simulink model "flat_model"  (R2023a)
settings: Solver=ode45  StartTime=0.0  StopTime=10.0  RelTol=1e-3  EnableMultiTasking=on
undefined symbols (not defined in the file): a0x, a0y, a0z, a1x, a1y, a1z, g, m
settings Model: Creator=Cesar Mtz  LastModifiedBy=20808
settings SolverCC: AlgebraicLoopSolver=TrustRegion
settings DataIOCC: LimitDataPoints=on  SaveFormat=Array  SignalLoggingSaveFormat=ModelDataLogs  ReturnWorkspaceOutputs=off
settings OptimizationCC: ExpressionDepthLimit=2147483647  LifeSpan=inf
settings DebuggingCC: UnderspecifiedInitializationDetection=Classic  MergeDetectMultiDrivingBlocksExec=none  SolverPrmCheckMsg=warning  FcnCallInpInsideContextMsg=warning  UnconnectedInputMsg=warning  UnconnectedOutputMsg=warning  UnconnectedLineMsg=warning  StateNameClashWarn=warning  SFUnexpectedBacktrackingDiag=warning  SFNoUnconditionalDefaultTransitionDiag=warning  SFExecutionAtInitializationDiag=none  ArithmeticOperatorsInVariantConditions=warning
settings HardwareCC: ProdBitPerPointer=32  ProdBitPerSizeT=32  ProdBitPerPtrDiffT=32  ProdLargestAtomicFloat=None  ProdIntDivRoundTo=Undefined  ProdEndianess=Unspecified  ProdWordSize=32  ProdHWDeviceType=32-bit Generic
settings ModelReferenceCC: EnableRefExpFcnMdlSchedulingChecks=on  PropagateSignalLabelsOutOfModel=off
settings SFSimCC: SimUseLocalCustomCode=off  CustomCodeUndefinedFunction=UseInterfaceOnly
settings RTWCC: RTWUseLocalCustomCode=off  DLArmComputeVersion=19.05
settings CodeAppCC: StateflowObjectComments=on
settings GRTTargetCC: TargetLangStandard=C89/C90 (ANSI)
settings ConfigComp: CovMetricSettings=dw  CovSaveCumulativeToWorkspaceVar=on  CovSaveSingleToWorkspaceVar=on  CovExternalEMLEnable=off

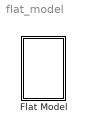
== system flat_model ==
  Flat Model : Subsystem

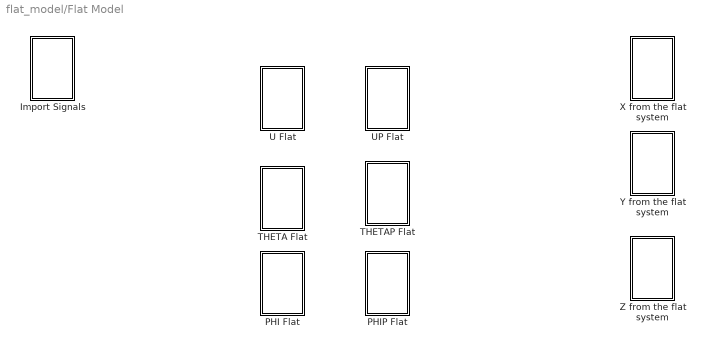
== system flat_model/Flat Model ==
  Import Signals : Subsystem
  PHI Flat : Subsystem
  PHIP Flat : Subsystem
  THETA Flat : Subsystem
  THETAP Flat : Subsystem
  U Flat : Subsystem
  UP Flat : Subsystem
  X from the flat system : Subsystem
  Y from the flat system : Subsystem
  Z from the flat system : Subsystem

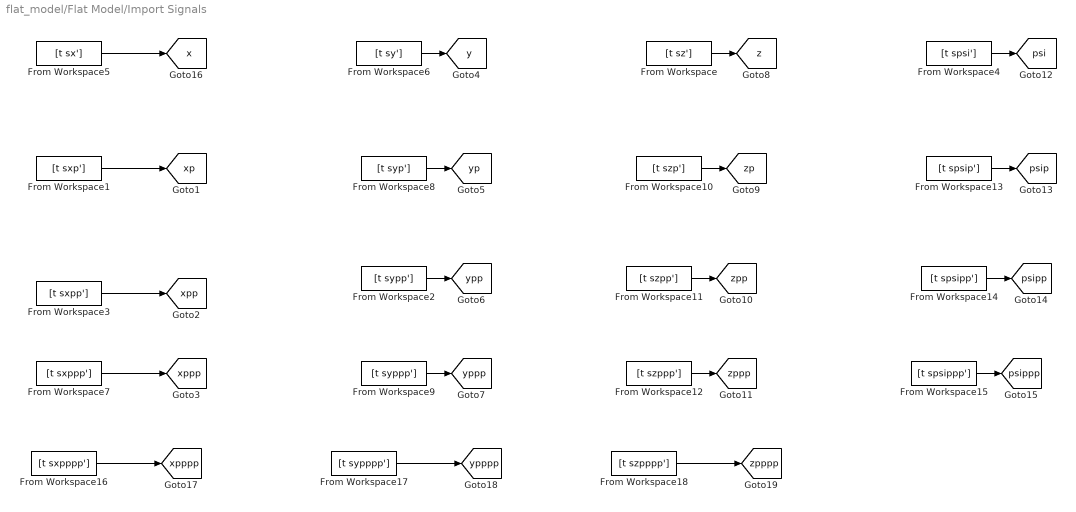
== system flat_model/Flat Model/Import Signals ==
  From Workspace : FromWorkspace  VariableName=[t sz']
  From Workspace1 : FromWorkspace  VariableName=[t sxp']
  From Workspace10 : FromWorkspace  VariableName=[t szp']
  From Workspace11 : FromWorkspace  VariableName=[t szpp']
  From Workspace12 : FromWorkspace  VariableName=[t szppp']
  From Workspace13 : FromWorkspace  VariableName=[t spsip']
  From Workspace14 : FromWorkspace  VariableName=[t spsipp']
  From Workspace15 : FromWorkspace  VariableName=[t spsippp']
  From Workspace16 : FromWorkspace  VariableName=[t sxpppp']
  From Workspace17 : FromWorkspace  VariableName=[t sypppp']
  From Workspace18 : FromWorkspace  VariableName=[t szpppp']
  From Workspace2 : FromWorkspace  VariableName=[t sypp']
  From Workspace3 : FromWorkspace  VariableName=[t sxpp']
  From Workspace4 : FromWorkspace  VariableName=[t spsi']
  From Workspace5 : FromWorkspace  VariableName=[t sx']  SampleTime=1
  From Workspace6 : FromWorkspace  VariableName=[t sy']
  From Workspace7 : FromWorkspace  VariableName=[t sxppp']
  From Workspace8 : FromWorkspace  VariableName=[t syp']
  From Workspace9 : FromWorkspace  VariableName=[t syppp']
  tag scope: psi=global, psip=global, psipp=global, psippp=global, x=global, xp=global, xpp=global, xppp=global, xpppp=global, y=global, yp=global, ypp=global, yppp=global, ypppp=global, z=global, zp=global, zpp=global, zppp=global, zpppp=global
  wires:
  From Workspace5/1 -> [x]
  From Workspace1/1 -> [xp]
  From Workspace3/1 -> [xpp]
  From Workspace7/1 -> [xppp]
  From Workspace6/1 -> [y]
  From Workspace8/1 -> [yp]
  From Workspace2/1 -> [ypp]
  From Workspace9/1 -> [yppp]
  From Workspace/1 -> [z]
  From Workspace10/1 -> [zp]
  From Workspace11/1 -> [zpp]
  From Workspace12/1 -> [zppp]
  From Workspace4/1 -> [psi]
  From Workspace13/1 -> [psip]
  From Workspace14/1 -> [psipp]
  From Workspace15/1 -> [psippp]
  From Workspace16/1 -> [xpppp]
  From Workspace17/1 -> [ypppp]
  From Workspace18/1 -> [zpppp]

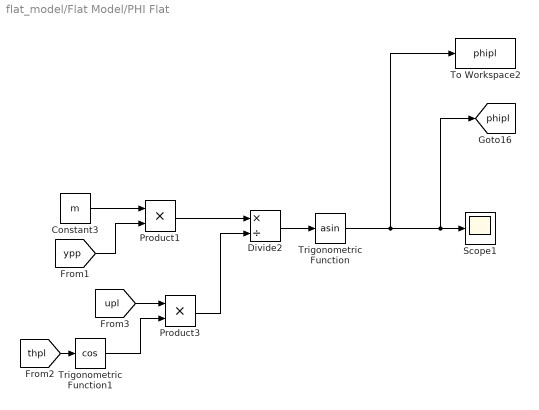
== system flat_model/Flat Model/PHI Flat ==
  Constant3 : Constant  Value=m
  Divide2 : Product  Inputs=*/
  Product1 : Product  RndMeth=Zero
  Product3 : Product  RndMeth=Zero
  Scope1 : Scope
  To Workspace2 : ToWorkspace  VariableName=phipl  SampleTime=-1
  Trigonometric Function : Trigonometry  Operator=asin
  Trigonometric Function1 : Trigonometry  Operator=cos
  tag scope: phipl=global
  wires:
  Product1/1 -> Divide2/1
  Divide2/1 -> Trigonometric Function/1
  [upl] -> Product3/1
  Trigonometric Function1/1 -> Product3/2
  Product3/1 -> Divide2/2
  Constant3/1 -> Product1/1
  [ypp] -> Product1/2
  Trigonometric Function/1 -> Scope1/1, [phipl], To Workspace2/1
  [thpl] -> Trigonometric Function1/1

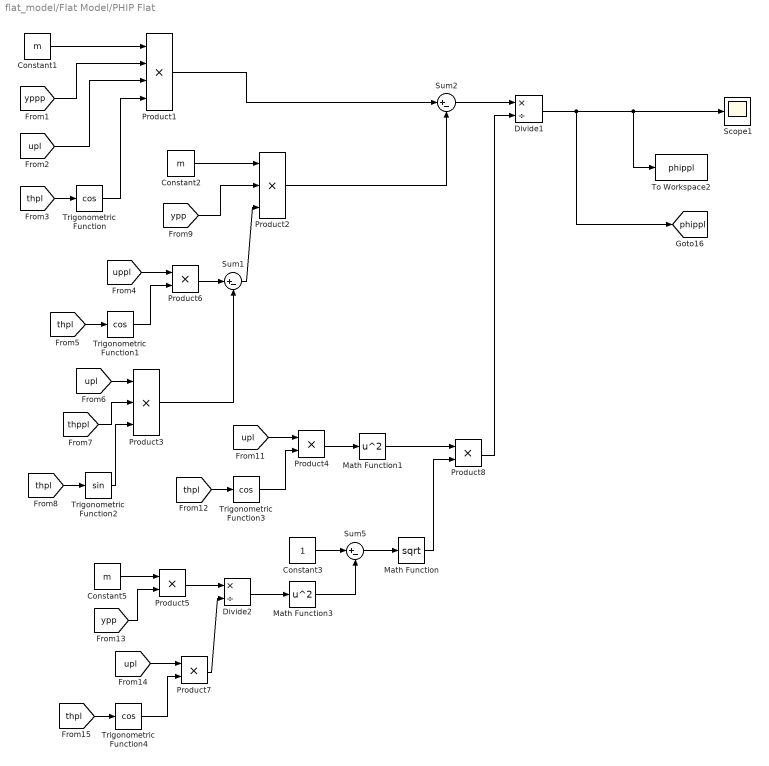
== system flat_model/Flat Model/PHIP Flat ==
  Constant1 : Constant  Value=m
  Constant2 : Constant  Value=m
  Constant3 : Constant
  Constant5 : Constant  Value=m
  Divide1 : Product  Inputs=*/
  Divide2 : Product  Inputs=*/
  Math Function : Math  Operator=sqrt  SignedPower=on
  Math Function1 : Math  Operator=square  SignedPower=on
  Math Function3 : Math  Operator=square  SignedPower=on
  Product1 : Product  Inputs=4  RndMeth=Zero
  Product2 : Product  Inputs=3  RndMeth=Zero
  Product3 : Product  Inputs=3  RndMeth=Zero
  Product{4..8} (5 alike) : Product  RndMeth=Zero
  Scope1 : Scope
  Sum1 : Sum  Inputs=|+-
  Sum2 : Sum  Inputs=|+-
  Sum5 : Sum  Inputs=|+-
  To Workspace2 : ToWorkspace  VariableName=phippl  SampleTime=-1
  Trigonometric Function{,1,3..4} (4 alike) : Trigonometry  Operator=cos
  Trigonometric Function2 : Trigonometry
  tag scope: phippl=global
  wires:
  Divide1/1 -> Scope1/1, To Workspace2/1, [phippl]
  Constant1/1 -> Product1/1
  [yppp] -> Product1/2
  [upl] -> Product1/3
  [thpl] -> Trigonometric Function/1
  Trigonometric Function/1 -> Product1/4
  [uppl] -> Product6/1
  [thpl] -> Trigonometric Function1/1
  Trigonometric Function1/1 -> Product6/2
  Product6/1 -> Sum1/1
  [upl] -> Product3/1
  [thppl] -> Product3/2
  [thpl] -> Trigonometric Function2/1
  Trigonometric Function2/1 -> Product3/3
  Product3/1 -> Sum1/2
  Constant2/1 -> Product2/1
  [ypp] -> Product2/2
  Sum1/1 -> Product2/3
  Product1/1 -> Sum2/1
  Product2/1 -> Sum2/2
  Sum2/1 -> Divide1/1
  [upl] -> Product4/1
  [thpl] -> Trigonometric Function3/1
  Trigonometric Function3/1 -> Product4/2
  Product4/1 -> Math Function1/1
  Constant5/1 -> Product5/1
  [ypp] -> Product5/2
  Product5/1 -> Divide2/1
  [upl] -> Product7/1
  [thpl] -> Trigonometric Function4/1
  Trigonometric Function4/1 -> Product7/2
  Product7/1 -> Divide2/2
  Divide2/1 -> Math Function3/1
  Constant3/1 -> Sum5/1
  Math Function3/1 -> Sum5/2
  Sum5/1 -> Math Function/1
  Math Function1/1 -> Product8/1
  Math Function/1 -> Product8/2
  Product8/1 -> Divide1/2

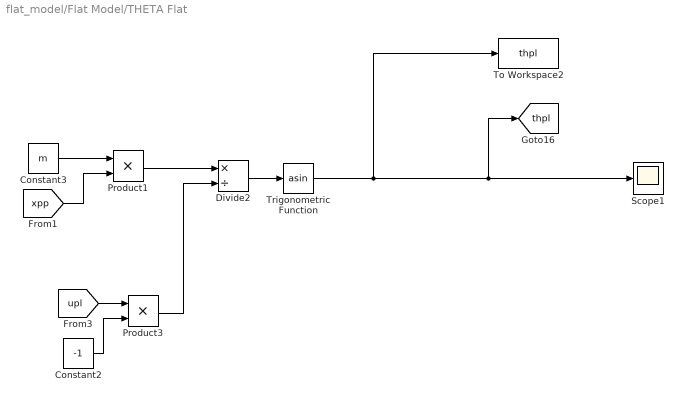
== system flat_model/Flat Model/THETA Flat ==
  Constant2 : Constant  Value=-1
  Constant3 : Constant  Value=m
  Divide2 : Product  Inputs=*/
  Product1 : Product  RndMeth=Zero
  Product3 : Product  RndMeth=Zero
  Scope1 : Scope
  To Workspace2 : ToWorkspace  VariableName=thpl  SampleTime=-1
  Trigonometric Function : Trigonometry  Operator=asin
  tag scope: thpl=global
  wires:
  Product1/1 -> Divide2/1
  Divide2/1 -> Trigonometric Function/1
  [upl] -> Product3/1
  Constant2/1 -> Product3/2
  Product3/1 -> Divide2/2
  Constant3/1 -> Product1/1
  [xpp] -> Product1/2
  Trigonometric Function/1 -> Scope1/1, [thpl], To Workspace2/1

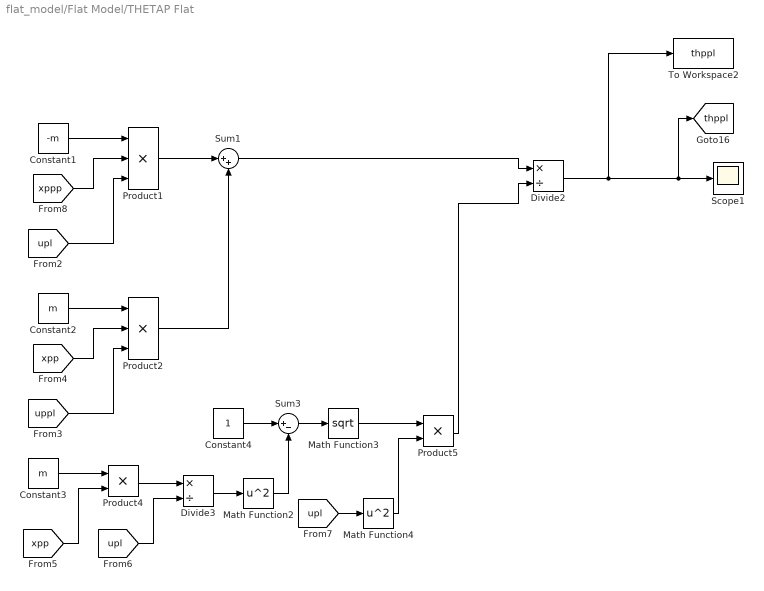
== system flat_model/Flat Model/THETAP Flat ==
  Constant1 : Constant  Value=-m
  Constant2 : Constant  Value=m
  Constant3 : Constant  Value=m
  Constant4 : Constant
  Divide2 : Product  Inputs=*/
  Divide3 : Product  Inputs=*/
  Math Function2 : Math  Operator=square  SignedPower=on
  Math Function3 : Math  Operator=sqrt  SignedPower=on
  Math Function4 : Math  Operator=square  SignedPower=on
  Product1 : Product  Inputs=3  RndMeth=Zero
  Product2 : Product  Inputs=3  RndMeth=Zero
  Product4 : Product  RndMeth=Zero
  Product5 : Product  RndMeth=Zero
  Scope1 : Scope
  Sum1 : Sum  Inputs=|++
  Sum3 : Sum  Inputs=|+-
  To Workspace2 : ToWorkspace  VariableName=thppl  SampleTime=-1
  tag scope: thppl=global
  wires:
  Constant1/1 -> Product1/1
  [xppp] -> Product1/2
  [upl] -> Product1/3
  Product1/1 -> Sum1/1
  Constant2/1 -> Product2/1
  [xpp] -> Product2/2
  [uppl] -> Product2/3
  Product2/1 -> Sum1/2
  Sum1/1 -> Divide2/1
  Product4/1 -> Divide3/1
  Constant3/1 -> Product4/1
  [xpp] -> Product4/2
  [upl] -> Divide3/2
  Divide3/1 -> Math Function2/1
  Constant4/1 -> Sum3/1
  Math Function2/1 -> Sum3/2
  Sum3/1 -> Math Function3/1
  Math Function3/1 -> Product5/1
  [upl] -> Math Function4/1
  Math Function4/1 -> Product5/2
  Product5/1 -> Divide2/2
  Divide2/1 -> Scope1/1, [thppl], To Workspace2/1

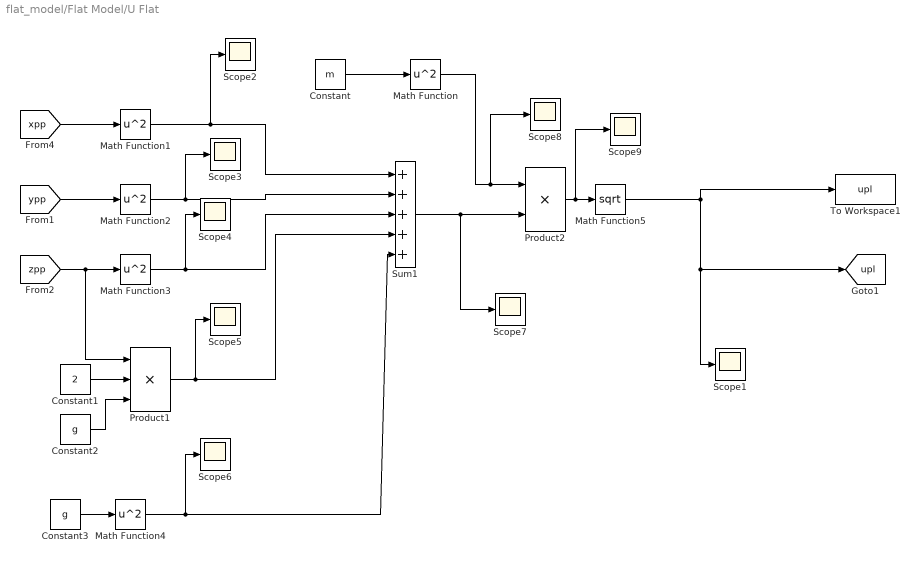
== system flat_model/Flat Model/U Flat ==
  Constant : Constant  Value=m
  Constant1 : Constant  Value=2
  Constant2 : Constant  Value=g
  Constant3 : Constant  Value=g
  Math Function{,1..4} (5 alike) : Math  Operator=square  SignedPower=on
  Math Function5 : Math  Operator=sqrt  SignedPower=on
  Product1 : Product  Inputs=3  RndMeth=Zero
  Product2 : Product  RndMeth=Zero
  Scope{1..9} (9 alike) : Scope
  Sum1 : Sum  Inputs=+++++
  To Workspace1 : ToWorkspace  VariableName=upl  SampleTime=-1
  tag scope: upl=global
  wires:
  Constant/1 -> Math Function/1
  [xpp] -> Math Function1/1
  [ypp] -> Math Function2/1
  [zpp] -> Math Function3/1, Product1/1
  Constant1/1 -> Product1/2
  Constant2/1 -> Product1/3
  Constant3/1 -> Math Function4/1
  Math Function1/1 -> Sum1/1, Scope2/1
  Math Function2/1 -> Sum1/2, Scope3/1
  Math Function3/1 -> Sum1/3, Scope4/1
  Product1/1 -> Sum1/4, Scope5/1
  Math Function4/1 -> Sum1/5, Scope6/1
  Math Function/1 -> Product2/1, Scope8/1
  Sum1/1 -> Product2/2, Scope7/1
  Product2/1 -> Math Function5/1, Scope9/1
  Math Function5/1 -> Scope1/1, [upl], To Workspace1/1

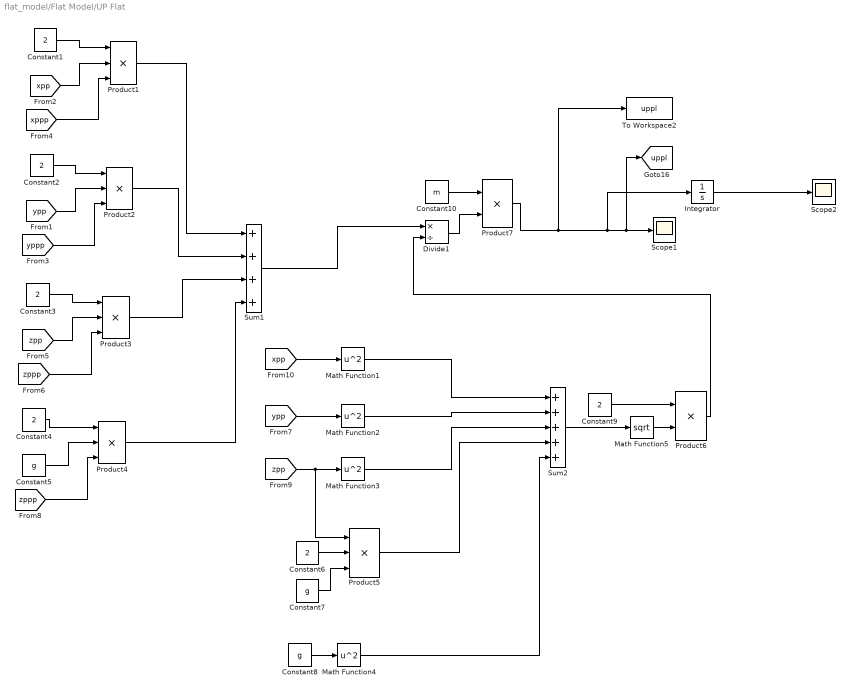
== system flat_model/Flat Model/UP Flat ==
  Constant{1..4,6,9} (6 alike) : Constant  Value=2
  Constant10 : Constant  Value=m
  Constant5 : Constant  Value=g
  Constant7 : Constant  Value=g
  Constant8 : Constant  Value=g
  Divide1 : Product  Inputs=*/
  Integrator : Integrator
  Math Function{1..4} (4 alike) : Math  Operator=square  SignedPower=on
  Math Function5 : Math  Operator=sqrt  SignedPower=on
  Product{1..5} (5 alike) : Product  Inputs=3  RndMeth=Zero
  Product6 : Product  RndMeth=Zero
  Product7 : Product  RndMeth=Zero
  Scope1 : Scope
  Scope2 : Scope
  Sum1 : Sum  Inputs=++++
  Sum2 : Sum  Inputs=+++++
  To Workspace2 : ToWorkspace  VariableName=uppl  SampleTime=-1
  tag scope: uppl=global
  wires:
  Constant1/1 -> Product1/1
  [xpp] -> Product1/2
  [xppp] -> Product1/3
  Constant2/1 -> Product2/1
  [ypp] -> Product2/2
  [yppp] -> Product2/3
  Constant3/1 -> Product3/1
  [zpp] -> Product3/2
  [zppp] -> Product3/3
  Constant4/1 -> Product4/1
  Constant5/1 -> Product4/2
  [zppp] -> Product4/3
  Product1/1 -> Sum1/1
  Product2/1 -> Sum1/2
  Product3/1 -> Sum1/3
  Product4/1 -> Sum1/4
  [xpp] -> Math Function1/1
  [ypp] -> Math Function2/1
  [zpp] -> Math Function3/1, Product5/1
  Constant6/1 -> Product5/2
  Constant7/1 -> Product5/3
  Constant8/1 -> Math Function4/1
  Math Function1/1 -> Sum2/1
  Math Function2/1 -> Sum2/2
  Math Function3/1 -> Sum2/3
  Product5/1 -> Sum2/4
  Math Function4/1 -> Sum2/5
  Sum2/1 -> Math Function5/1
  Constant9/1 -> Product6/1
  Math Function5/1 -> Product6/2
  Constant10/1 -> Product7/1
  Divide1/1 -> Product7/2
  Sum1/1 -> Divide1/1
  Product6/1 -> Divide1/2
  Product7/1 -> To Workspace2/1, Scope1/1, [uppl], Integrator/1
  Integrator/1 -> Scope2/1

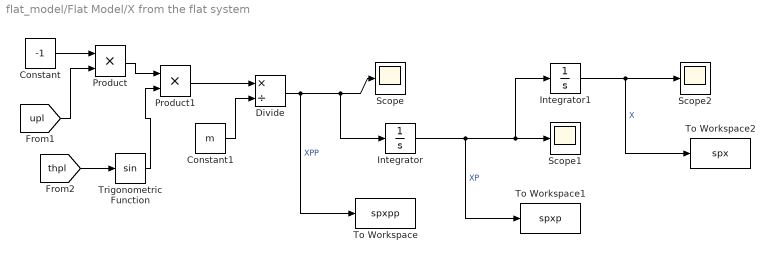
== system flat_model/Flat Model/X from the flat system ==
  Constant : Constant  Value=-1
  Constant1 : Constant  Value=m
  Divide : Product  Inputs=*/
  Integrator : Integrator  InitialCondition=a1x
  Integrator1 : Integrator  InitialCondition=a0x
  Product : Product  RndMeth=Zero
  Product1 : Product  RndMeth=Zero
  Scope : Scope
  Scope1 : Scope
  Scope2 : Scope
  To Workspace : ToWorkspace  VariableName=spxpp  SampleTime=-1
  To Workspace1 : ToWorkspace  VariableName=spxp  SampleTime=-1
  To Workspace2 : ToWorkspace  VariableName=spx  SampleTime=-1
  Trigonometric Function : Trigonometry
  wires:
  Constant/1 -> Product/1
  [upl] -> Product/2
  Product/1 -> Product1/1
  Trigonometric Function/1 -> Product1/2
  [thpl] -> Trigonometric Function/1
  Product1/1 -> Divide/1
  Constant1/1 -> Divide/2
  Divide/1 -> Scope/1, Integrator/1, To Workspace/1  "XPP"
  Integrator/1 -> Scope1/1, Integrator1/1, To Workspace1/1  "XP"
  Integrator1/1 -> Scope2/1, To Workspace2/1  "X"

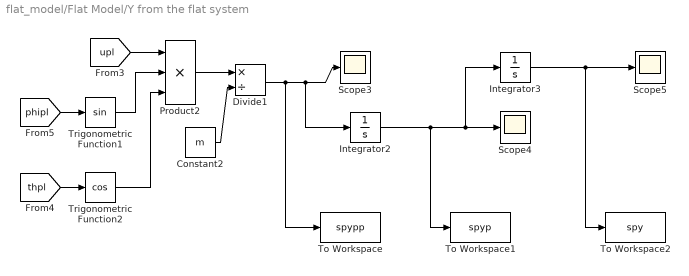
== system flat_model/Flat Model/Y from the flat system ==
  Constant2 : Constant  Value=m
  Divide1 : Product  Inputs=*/
  Integrator2 : Integrator  InitialCondition=a1y
  Integrator3 : Integrator  InitialCondition=a0y
  Product2 : Product  Inputs=3  RndMeth=Zero
  Scope3 : Scope
  Scope4 : Scope
  Scope5 : Scope
  To Workspace : ToWorkspace  VariableName=spypp  SampleTime=-1
  To Workspace1 : ToWorkspace  VariableName=spyp  SampleTime=-1
  To Workspace2 : ToWorkspace  VariableName=spy  SampleTime=-1
  Trigonometric Function1 : Trigonometry
  Trigonometric Function2 : Trigonometry  Operator=cos
  wires:
  [upl] -> Product2/1
  Trigonometric Function1/1 -> Product2/2
  Trigonometric Function2/1 -> Product2/3
  [thpl] -> Trigonometric Function2/1
  [phipl] -> Trigonometric Function1/1
  Product2/1 -> Divide1/1
  Constant2/1 -> Divide1/2
  Divide1/1 -> Integrator2/1, Scope3/1, To Workspace/1
  Integrator2/1 -> Integrator3/1, Scope4/1, To Workspace1/1
  Integrator3/1 -> Scope5/1, To Workspace2/1

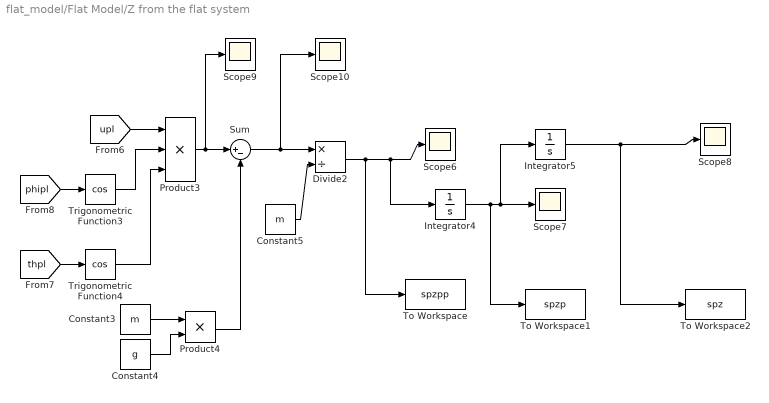
== system flat_model/Flat Model/Z from the flat system ==
  Constant3 : Constant  Value=m
  Constant4 : Constant  Value=g
  Constant5 : Constant  Value=m
  Divide2 : Product  Inputs=*/
  Integrator4 : Integrator  InitialCondition=a1z
  Integrator5 : Integrator  InitialCondition=a0z
  Product3 : Product  Inputs=3  RndMeth=Zero
  Product4 : Product  RndMeth=Zero
  Scope{6..10} (5 alike) : Scope
  Sum : Sum  Inputs=|+-
  To Workspace : ToWorkspace  VariableName=spzpp  SampleTime=-1
  To Workspace1 : ToWorkspace  VariableName=spzp  SampleTime=-1
  To Workspace2 : ToWorkspace  VariableName=spz  SampleTime=-1
  Trigonometric Function3 : Trigonometry  Operator=cos
  Trigonometric Function4 : Trigonometry  Operator=cos
  wires:
  [upl] -> Product3/1
  Trigonometric Function3/1 -> Product3/2
  Trigonometric Function4/1 -> Product3/3
  [thpl] -> Trigonometric Function4/1
  [phipl] -> Trigonometric Function3/1
  Product3/1 -> Sum/1, Scope9/1
  Product4/1 -> Sum/2
  Constant3/1 -> Product4/1
  Constant4/1 -> Product4/2
  Sum/1 -> Divide2/1, Scope10/1
  Constant5/1 -> Divide2/2
  Divide2/1 -> Scope6/1, Integrator4/1, To Workspace/1
  Integrator4/1 -> Scope7/1, Integrator5/1, To Workspace1/1
  Integrator5/1 -> Scope8/1, To Workspace2/1
